simulink model "Prep_Matlab2_P10"  (R2024b)
settings: Solver=VariableStepAuto  StartTime=0.0  StopTime=50  RelTol=1e-3
settings Model: Creator=yviki  LastModifiedBy=simon
settings DebuggingCC: UnconnectedInputMsg=warning  UnconnectedOutputMsg=warning  UnconnectedLineMsg=warning
settings ModelReferenceCC: EnableRefExpFcnMdlSchedulingChecks=on
settings RTWCC: GPUComputeCapability=3.5  DLArmComputeVersion=19.05

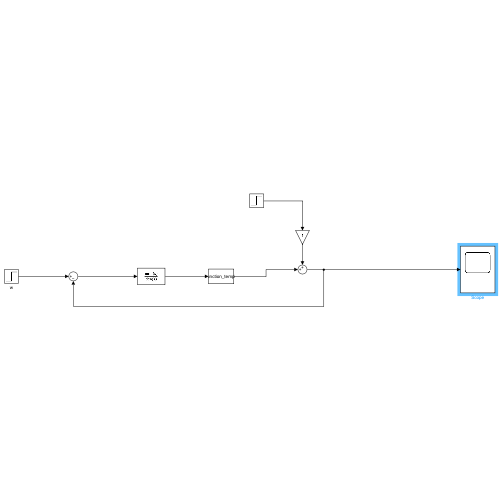
[thumbnail: Simulink's stored preview of the top-level diagram]
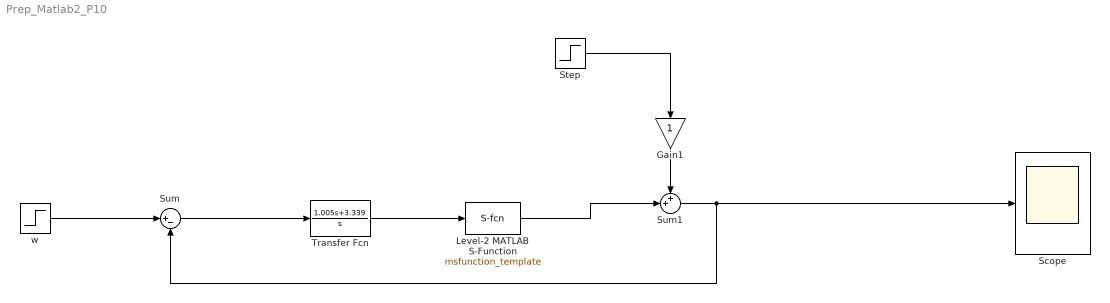
== system Prep_Matlab2_P10 ==
  Gain1 : Gain
  Level-2 MATLAB S-Function : M-S-Function  FunctionName=msfunction_template  Parameters=[-1;-1]
  Scope : Scope
  Step : Step  SampleTime=0
  Sum : Sum  Inputs=|+-
  Sum1 : Sum  Inputs=++|
  Transfer Fcn : TransferFcn  Numerator=[1.005 3.339]  Denominator=[1 0]
  w : Step  After=0.79  SampleTime=0
  wires:
  Sum1/1 -> Sum/2, Scope/1
  Gain1/1 -> Sum1/1
  Step/1 -> Gain1/1
  w/1 -> Sum/1
  Level-2 MATLAB S-Function/1 -> Sum1/2
  Sum/1 -> Transfer Fcn/1
  Transfer Fcn/1 -> Level-2 MATLAB S-Function/1
